simulink model "test12"  (R2024a)
settings: Solver=FixedStepAuto  StartTime=0.0  StopTime=30  FixedStep=0.001  MaxStep=1e-2  RelTol=1e-3
libraries: fl_lib x21, nesl_utility x14, sdl_lib x8, simulink x4
(part 1 of 2)
settings Model: DataDictionary=test4.sldd  Creator=18311  LastModifiedBy=18311

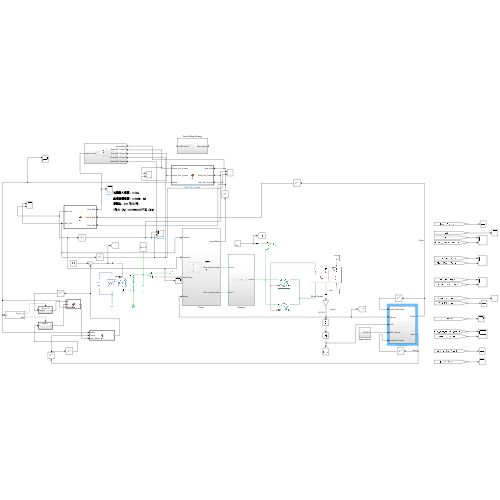
[thumbnail: Simulink's stored preview of the top-level diagram]
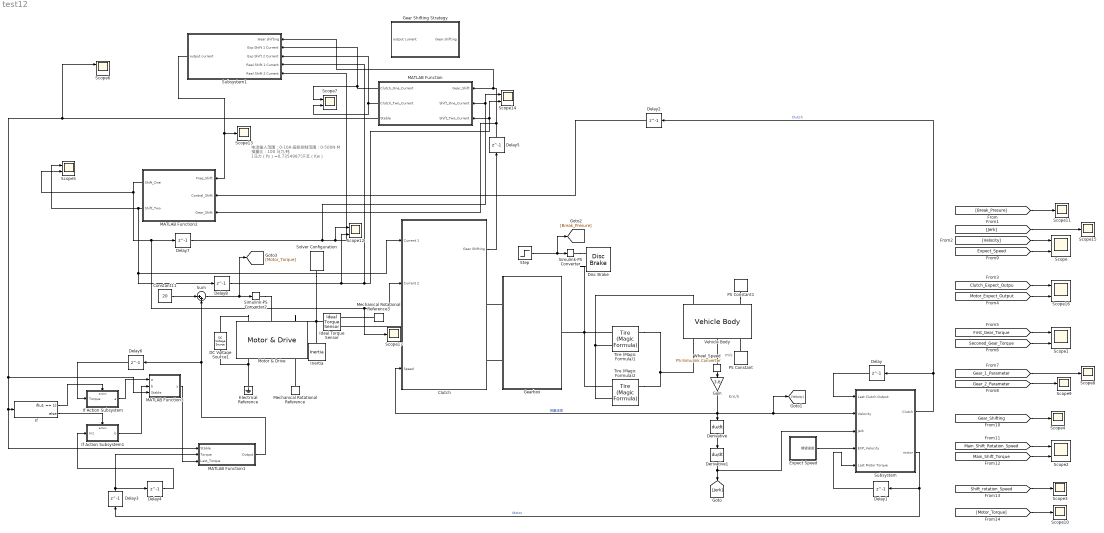
== system test12 ==
  note: Km/h
  note: m/s
  note: 电流输入范围：0-10A
      | 扭矩控制范围：0-500N·M
      | 推重比：100 马力/吨
      | 1马力（Ps）=0.73549875千瓦（Kw）
  Clutch : Subsystem
      settings: PortSchema="{\"entries\":[{\"content\":{\"sides\":[{\"content\":{\"connectorIds\":[\"In1\",\"In2\",\"LConn1\",\"In3\"]},\"type\":\"ConnectorPlacement.EquallySpacedRectSide\",\"uuid\":\"056ad525-3a8f-4273-b105-de9e991d8580\"},{\"content\":{\"connectorIds\":[\"Out1\",\"RConn1\",\"RConn2\"],\"side\":\"RIGHT\"},\"type\":\"ConnectorPlacement.EquallySpacedRectSide\",\"uuid\":\"78f39029-2d72-4f9a-95da-9e6af56cb8b6\"},{\"content\":{\"side\":\"TOP\"},\"type\":\"ConnectorPlacement.EquallySpacedRectSide\",\"uuid\":\"380b0431-6fdd-4cff-97a6-25de2baed91e\"}]},\"type\":\"ConnectorPlacement.EquallySpacedConnector\",\"uuid\":\"d5c6ad5a-c539-4d45-a449-cd47a7a8a4ab\"}],\"packageUris\":[\"http://schema.mathworks.com/mf0/Connector/R2020b\"],\"version\":\"1.0\"}"
  Constant11 : Constant  Value=20
  DC Voltage Source1 : fl_lib/Electrical/Electrical Sources/DC Voltage Source  v0=220 V
  Delay{,1..8} (9 alike) : Delay  DelayLength=1  InitialCondition=0
  Derivative : Derivative
  Derivative1 : Derivative
  Disc Brake : sdl_lib/Brakes & Detents/Rotational/Disc Brake  r_mean=150 mm  bore=10 mm  n_pads=2  enable_faults=simscape.enum.onoff.off  faulted_pressure=0 bar  thermal_port=simscape.enum.thermaleffects.omit  mu_static=0.9  mu_coulomb=0.7  temperature_TLU=[280, 300, 320] K  mu_static_TLU=[.9, .8, .7]  mu_coulomb_TLU=[.8, .7, .6]  brkwy_vel=0.1 rad/s  visc_coef=0 N*m*s/rad  thermal_mass=50 kJ/K  temperature_specify=off  temperature_priority=High  temperature=300 K  temperature_nominal_specify=off  temperature_nominal_value=1  temperature_nominal_unit=K
  Electrical Reference : fl_lib/Electrical/Electrical Elements/Electrical Reference
  Expect Speed : Subsystem
  Gain : Gain  Gain=3.6
  Gear Shifting Strategy : Subsystem
  Gearbox : Subsystem
  Ideal Torque Sensor : fl_lib/Mechanical/Mechanical Sensors/Ideal Torque Sensor
  If : If  IfExpression=u1 == 1
  If Action Subsystem : Subsystem  TreatAsAtomicUnit=on
  If Action Subsystem1 : Subsystem  TreatAsAtomicUnit=on
  Inertia : fl_lib/Mechanical/Rotational Elements/Inertia  inertia=0.01 kg*m^2  num_ports=foundation.enum.numPorts2.one  w_specify=off  w_priority=High  w=0 rad/s  w_nominal_specify=off  w_nominal_value=1  w_nominal_unit=rad/s  t_specify=off  t_priority=None  t=0 N*m  t_nominal_specify=off  t_nominal_value=1  t_nominal_unit=N*m
  MATLAB Function : MATLAB Function  TreatAsAtomicUnit=on
  MATLAB Function1 : MATLAB Function  TreatAsAtomicUnit=on
  MATLAB Function2 : MATLAB Function  TreatAsAtomicUnit=on
  MATLAB Function3 : MATLAB Function  TreatAsAtomicUnit=on
  Mechanical Rotational Reference : fl_lib/Mechanical/Rotational Elements/Mechanical Rotational Reference
  Mechanical Rotational Reference3 : fl_lib/Mechanical/Rotational Elements/Mechanical Rotational Reference
  Motor & Drive : sdl_lib/Engines & Motors/Motor & Drive  torque_max=200 N*m  power_max=73.549875 kW  Tc=0.02 s  eff=100  w_eff=4000 rpm  T_eff=200 N*m  thermal_port=simscape.enum.thermaleffects.omit  thermal_mass=100 J/K  temperature_specify=off  temperature_priority=High  temperature=300 K  temperature_nominal_specify=off  temperature_nominal_value=1  temperature_nominal_unit=K
      settings: InternalSimscapePortConfiguration="{\"Bottom\":[],\"Left\":[{\"id\":\"Vp\",\"label\":\"+\",\"type\":\"foundation.electrical.electrical\"},{\"id\":\"Tr\",\"label\":\"Tr\",\"type\":\"input\"},{\"id\":\"R\",\"label\":\"R\",\"type\":\"foundation.mechanical.rotational.rotational\"}],\"Right\":[{\"id\":\"Vm\",\"label\":\"-\",\"type\":\"foundation.electrical.electrical\"},{\"id\":\"Omega\",\"label\":\"w\",\"type\":\"output\"},{\"id\":\"C\",\"label\":\"C\",\"type\":\"foundation.mechanical.rotational.rotational\"}],\"Top\":[]}"
  PS Constant : fl_lib/Physical Signals/Sources/PS Constant  constant=0
  PS Constant1 : fl_lib/Physical Signals/Sources/PS Constant  constant=0
  Scope{,1..2,5..7,12,14,16} (9 alike) : Scope  NumInputPorts=2
  Scope{3..4,8..11,13,15,17} (9 alike) : Scope
  Simulink-PS Converter : nesl_utility/Simulink-PS Converter  PhysicalDomain=network_engine_domain  SubClassName=ps_input  LeftPortType=input  RightPortType=output  PseudoPeriodic=off  Frequencies=[]  NoiseDistribution=none  NoiseParameters=[]  Unit=1  AffineConversion=off  FilteringAndDerivatives=provide  SimscapeFilterOrder=1  InputFilterTimeConstant=0.001  UdotUserProvided=0
  Simulink-PS Converter2 : nesl_utility/Simulink-PS Converter  PhysicalDomain=network_engine_domain  SubClassName=ps_input  LeftPortType=input  RightPortType=output  PseudoPeriodic=off  Frequencies=[]  NoiseDistribution=none  NoiseParameters=[]  Unit=1  AffineConversion=off  FilteringAndDerivatives=provide  SimscapeFilterOrder=1  InputFilterTimeConstant=0.001  UdotUserProvided=0
  Solver Configuration : nesl_utility/Solver Configuration  PhysicalDomain=network_engine_domain  SubClassName=solver  LeftPortType=input  RightPortType=generic  Tones=[]  Harmonics=[]  SimulateNoise=off  Profile=off  UseLocalSampling=off  EnableSwitchedLinearOptims=on  FrequencyDomain=off  UseCCode=off  RelTol=0.001  AbsTol=0.001  MinStep=1e-09  ToWorkspace=off  RevertToSquareIcSolve=off  NumHomotopyIterations=100  PhasorMode=off  PhasorModeNumHarmonics=1  ConsistencySolver=NEWTON_XTOL_AFTER_FTOL  IndexReductionMethod=DerivativeReplacement  DoDC=off  ResidualTolerance=1e-09  ConsistencyTolSource=GLOBAL  ConsistencyAbsTol=0.001  ConsistencyRelTol=0.001  ConsistencyTolFactor=0.001  UseLocalSolver=off  LocalSolverChoice=NE_BACKWARD_EULER_ADVANCER  ResolveIndetEquations=on  FunctionEvalNumThread=1  LocalSolverSampleTime=0.001  DoFixedCost=off  MaxNonlinIter=3  MaxModeIter=2  ComputeImpulses=off  ImpulseIterations=2  LinearAlgebra=auto  LinearAlgebraNumThread=0  EquationFormulation=NE_TIME_EF  DelaysMemoryBudget=1024  AutomaticFiltering=on  FilteringTimeConstant=0.001  PartitionStorageMethod=AS_NEEDED  PartitionMemoryBudget=1024  PartitionMethod=ROBUST  MultibodyUseLocalSolver=off  MultibodyLocalSolverChoice=ODE1  MultibodyLocalSolverSampleTime=0.001
  Step : Step  Time=20  After=150  SampleTime=0
  Subsystem : Subsystem
  Subsystem1 : Subsystem
  Sum : Sum  Inputs=|++
  Tire (Magic Formula)1 : sdl_lib/Tires & Vehicles/Tire (Magic Formula)  parameterization=sdl.enum.magic_tire_model.peak  F_z1=2500 N  F_x1=3500 N  kappa1=10  B_m=10  C_m=1.9  D_m=1  E_m=0.97  fz0=4000 N  p_Cx=1.685  p_Dx=[1.21, -.037]  p_Ex=[.344, .095, -.02, 0]  p_Kx=[21.51, -.163, .245]  p_Hx=[-.002, .002]  p_Vx=[0, 0]  rolling_radius_model=sdl.enum.RollingRadiusParameterization.Constant  r_e=0.3 m  r_0=0.3 m  breff=8.39  dreff=0.26  freff=0.074  q_re0=0.99  q_v1=0.008  longvl=17 m/s  cz=5e5 N/m  model_resistance=true  resistance_model=sdl.enum.rollingResistanceParameterization.constant  coeff=0.015  p_tire=250e3 Pa  alpha=-0.003  beta=0.97  coeff_a=84e-4  coeff_b=6.2e-4 s/m  coeff_c=1.6e-4 s^2/m^2  p_tire0=240e3 Pa  fz0_resistance=4000 N  vH0=16 m/s  q_Sy=[.0082, 0, .0014, .001, 0, 0, 1.08, -.5]  v_thr=0.001 m/s  enable_scaling_coefficients=false  lfzO=1  lcx=1  lmux=1  lex=1  lkx=1  lhx=1  lvx=1  lmy=1  model_compliance=sdl.enum.compliance.off  stiffness=1e6 N/m  damping=1000 N*s/m  model_inertia=sdl.enum.model_inertia.off  inertia=1 kg*m^2  initial_velocity=0 rad/s  vxlow=1 m/s  v_tr_thr=0.1 m/s  kpumin=-1.5  kpumax=1.5
  Tire (Magic Formula)2 : sdl_lib/Tires & Vehicles/Tire (Magic Formula)  parameterization=sdl.enum.magic_tire_model.peak  F_z1=2500 N  F_x1=3000 N  kappa1=10  B_m=10  C_m=1.9  D_m=1  E_m=0.97  fz0=4000 N  p_Cx=1.685  p_Dx=[1.21, -.037]  p_Ex=[.344, .095, -.02, 0]  p_Kx=[21.51, -.163, .245]  p_Hx=[-.002, .002]  p_Vx=[0, 0]  rolling_radius_model=sdl.enum.RollingRadiusParameterization.Constant  r_e=0.3 m  r_0=0.3 m  breff=8.39  dreff=0.26  freff=0.074  q_re0=0.99  q_v1=0.008  longvl=17 m/s  cz=5e5 N/m  model_resistance=true  resistance_model=sdl.enum.rollingResistanceParameterization.constant  coeff=0.015  p_tire=250e3 Pa  alpha=-0.003  beta=0.97  coeff_a=84e-4  coeff_b=6.2e-4 s/m  coeff_c=1.6e-4 s^2/m^2  p_tire0=240e3 Pa  fz0_resistance=4000 N  vH0=16 m/s  q_Sy=[.0082, 0, .0014, .001, 0, 0, 1.08, -.5]  v_thr=0.001 m/s  enable_scaling_coefficients=false  lfzO=1  lcx=1  lmux=1  lex=1  lkx=1  lhx=1  lvx=1  lmy=1  model_compliance=sdl.enum.compliance.off  stiffness=1e6 N/m  damping=1000 N*s/m  model_inertia=sdl.enum.model_inertia.off  inertia=1 kg*m^2  initial_velocity=0 rad/s  vxlow=1 m/s  v_tr_thr=0.1 m/s  kpumin=-1.5  kpumax=1.5
  Vehicle Body : sdl_lib/Tires & Vehicles/Vehicle Body  mass=1000 kg  n_w=1  x_f=1.4 m  x_r=1.6 m  y_c=0.5 m  mass_var=simscape.enum.onoff.off  g=9.81 m/s^2  liftoff_warning=simscape.enum.onoff.off  area=3 m^2  Cd=0.4  rho=1.18 kg/m^3  model_pitch=simscape.enum.onoff.off  inertia=4000 kg*m^2  suspension_model=sdl.enum.linearTLU.linear  k_f=1e4 N/m  b_f=1e4 N*s/m  k_r=1e4 N/m  b_r=1e4 N*s/m  k_f_TLU=[-2000, -1000, 0, 1000, 2000] N  x_f_TLU=[-.4, -.2, 0, .2, .4] m  b_f_TLU=[-200, -100, 0, 100, 200] N  v_f_TLU=[-4, -2, 0, 2, 4] m/s  k_r_TLU=[-2000, -1000, 0, 1000, 2000] N  x_r_TLU=[-.4, -.2, 0, .2, .4] m  b_r_TLU=[-200, -100, 0, 100, 200] N  v_r_TLU=[-4, -2, 0, 2, 4] m/s  interp_method=simscape.enum.interpolation.linear  extrap_method=simscape.enum.extrapolation.linear  model_hardstop=simscape.enum.onoff.off  upper_bound_f=.25 m  lower_bound_f=-.25 m  stop_k_f=1e6 N/m  stop_b_f=150 N*s/m  upper_bound_r=.25 m  lower_bound_r=-.25 m  stop_k_r=1e6 N/m  stop_b_r=150 N*s/m  initial_pitch=0 rad  initial_pitch_rate=0 rad/s  v_specify=off  v_priority=High  v=0 m/s  v_nominal_specify=off  v_nominal_value=1  v_nominal_unit=m/s
  Wheel_Speed : nesl_utility/PS-Simulink Converter  PhysicalDomain=network_engine_domain  SubClassName=ps_output  LeftPortType=input  RightPortType=output  PseudoPeriodic=off  Frequencies=[]  VectorFormat=inherit  Unit=inherit  AffineConversion=off
  wires:
  Wheel_Speed/1 -> Gain/1
  Derivative/1 -> Derivative1/1
  Constant11/1 -> Sum/1
  Sum/1 -> [Motor_Torque], Simulink-PS Converter2/1
  Subsystem/2(motor) -> Delay1/1, Delay3/1  "Motor"
  Subsystem/1(Clutch) -> Delay2/1, Delay/1  "Clutch"
  Gain/1 -> Derivative/1, [Velocity], Subsystem/2(Velocity), Clutch/3(Speed)  "测量速度"
  Clutch/1(Gear Shifting) -> Delay5/1
  Expect Speed/1(期望速度) -> Subsystem/4(EXP_Velocity)
  Delay/1 -> Subsystem/1(Last Clutch Output)
  Delay1/1 -> Subsystem/5(Last Motor Torque)
  Derivative1/1 -> [Jerk], Subsystem/3(Jerk)
  [Velocity] -> Scope/1
  [Expect_Speed] -> Scope/2
  [First_Gear_Torque] -> Scope1/1
  [Seconed_Gear_Torque] -> Scope1/2
  [Main_Shift_Torque] -> Scope2/2
  [Main_Shift_Rotation_Speed] -> Scope2/1
  [Shift_rotation_Speed] -> Scope3/1
  Delay5/1 -> MATLAB Function2/3(Gear_Shift), Subsystem1/1(Gear shifting), MATLAB Function/1(Gear_Shift)
  If/1 -> If Action Subsystem/Action
  If/2 -> If Action Subsystem1/Action
  MATLAB Function/3(Stable) -> Scope6/1, MATLAB Function3/3(Stable), MATLAB Function1/1(Stable), If/1
  Delay3/1 -> MATLAB Function1/2(Torque), Delay4/1
  MATLAB Function1/1(Output) -> Delay6/1, Sum/2
  Delay4/1 -> If Action Subsystem1/1(In1)
  Delay6/1 -> If Action Subsystem/1(Torque)
  MATLAB Function3/1(y) -> MATLAB Function1/3(Last_Torque)
  If Action Subsystem/1(a) -> MATLAB Function3/1(a)
  If Action Subsystem1/1(b) -> MATLAB Function3/2(b)
  MATLAB Function/1(Clutch_One_Current) -> Subsystem1/2(Exp Shift 1 Current), Scope7/1
  MATLAB Function/2(Clutch_Two_Current) -> Subsystem1/3(Exp Shift 2 Current), Scope7/2
  Delay2/1 -> MATLAB Function2/2(Contral_Shift)
  Subsystem1/1(output current) -> Scope13/1, MATLAB Function2/1(Free_Shift)
  MATLAB Function2/1(Shift_One) -> Scope5/2, Clutch/2(Current 2), Scope17/1, Delay7/1
  MATLAB Function2/2(Shift_Two) -> Scope5/1, Delay8/1, Clutch/1(Current 1)
  [Gear_Shifting] -> Scope4/1
  Delay7/1 -> Subsystem1/5(Real Shift 2 Current), Scope12/1, Scope14/1, MATLAB Function/2(Shift_One_Current)
  Delay8/1 -> Subsystem1/4(Real Shift 1 Current), Scope14/2, MATLAB Function/3(Shift_Two_Current), Scope12/2
  [Gear_1_Parameter] -> Scope8/1
  [Gear_2_Parameter] -> Scope9/1
  [Motor_Torque] -> Scope10/1
  [Break_Presure] -> Scope11/1
  Step/1 -> [Break_Presure], Simulink-PS Converter/1
  [Jerk] -> Scope15/1
  [Clutch_Expect_Outpu] -> Scope16/1
  [Motor_Expect_Output] -> Scope16/2
  connections:
  Motor & Drive/LConn1 -- DC Voltage Source1/LConn1
  Electrical Reference/LConn1 -- DC Voltage Source1/RConn1 -- Motor & Drive/RConn1
  Mechanical Rotational Reference/LConn1 -- Motor & Drive/RConn3
  Inertia/LConn1 -- Motor & Drive/LConn3 -- Solver Configuration/RConn1 -- Ideal Torque Sensor/LConn1
  PS Constant/RConn1 -- Vehicle Body/LConn3
  PS Constant1/RConn1 -- Vehicle Body/RConn3
  Clutch/LConn1 -- Ideal Torque Sensor/RConn2
  Wheel_Speed/LConn1 -- Vehicle Body/LConn2
  Simulink-PS Converter2/RConn1 -- Motor & Drive/LConn2
  Tire (Magic Formula)1/RConn2 -- Tire (Magic Formula)2/RConn2 -- Vehicle Body/LConn1
  Tire (Magic Formula)1/LConn1 -- Tire (Magic Formula)2/LConn1 -- Vehicle Body/RConn1
  Mechanical Rotational Reference3/LConn1 -- Ideal Torque Sensor/RConn1
  Simulink-PS Converter/RConn1 -- Disc Brake/LConn1
  Disc Brake/LConn2 -- Tire (Magic Formula)1/LConn2 -- Tire (Magic Formula)2/LConn2 -- Gearbox/RConn1
  Gearbox/LConn1 -- Clutch/RConn1
  Gearbox/LConn2 -- Clutch/RConn2

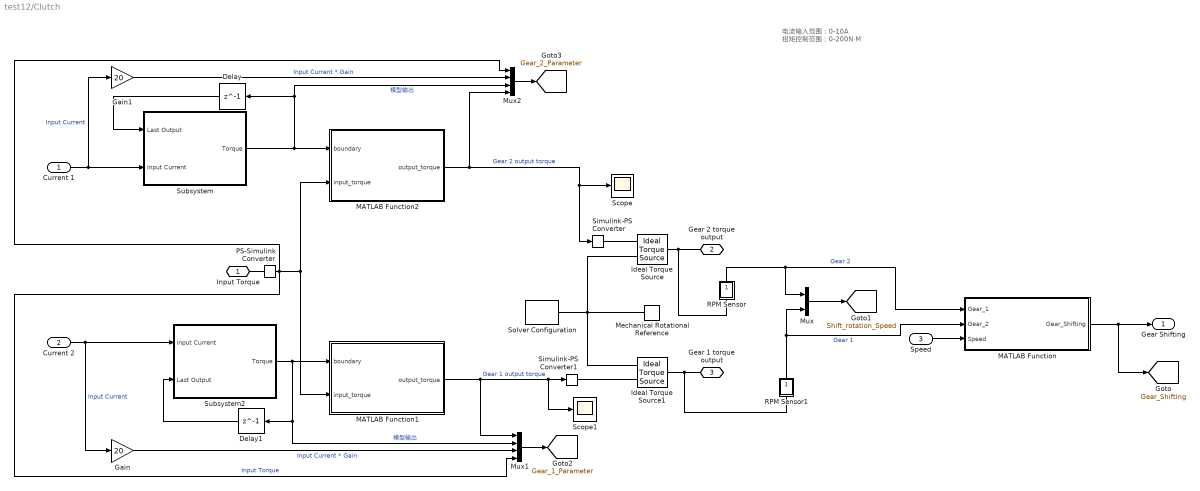
== system test12/Clutch ==
  note: 电流输入范围：0-10A
      | 扭矩控制范围：0-200N·M
  Current 1 : Inport
  Current 2 : Inport  Port=2
  Speed : Inport  Port=3
  Delay : Delay  DelayLength=1  InitialCondition=0
  Delay1 : Delay  DelayLength=1  InitialCondition=0
  Gain : Gain  Gain=20
  Gain1 : Gain  Gain=20
  Ideal Torque Source : fl_lib/Mechanical/Mechanical Sources/Ideal Torque Source
  Ideal Torque Source1 : fl_lib/Mechanical/Mechanical Sources/Ideal Torque Source
  MATLAB Function : MATLAB Function  TreatAsAtomicUnit=on
  MATLAB Function1 : MATLAB Function  TreatAsAtomicUnit=on
  MATLAB Function2 : MATLAB Function  TreatAsAtomicUnit=on
  Mechanical Rotational Reference : fl_lib/Mechanical/Rotational Elements/Mechanical Rotational Reference
  Mux : Mux  Inputs=2
  Mux1 : Mux
  Mux2 : Mux
  PS-Simulink Converter : nesl_utility/PS-Simulink Converter  PhysicalDomain=network_engine_domain  SubClassName=ps_output  LeftPortType=input  RightPortType=output  PseudoPeriodic=off  Frequencies=[]  VectorFormat=inherit  Unit=inherit  AffineConversion=off
  RPM Sensor : Subsystem
      mask Display: disp('S')
  RPM Sensor1 : Subsystem
      mask Display: disp('S')
  Scope : Scope
  Scope1 : Scope
  Simulink-PS Converter : nesl_utility/Simulink-PS Converter  PhysicalDomain=network_engine_domain  SubClassName=ps_input  LeftPortType=input  RightPortType=output  PseudoPeriodic=off  Frequencies=[]  NoiseDistribution=none  NoiseParameters=[]  Unit=1  AffineConversion=off  FilteringAndDerivatives=provide  SimscapeFilterOrder=1  InputFilterTimeConstant=0.001  UdotUserProvided=0
  Simulink-PS Converter1 : nesl_utility/Simulink-PS Converter  PhysicalDomain=network_engine_domain  SubClassName=ps_input  LeftPortType=input  RightPortType=output  PseudoPeriodic=off  Frequencies=[]  NoiseDistribution=none  NoiseParameters=[]  Unit=1  AffineConversion=off  FilteringAndDerivatives=provide  SimscapeFilterOrder=1  InputFilterTimeConstant=0.001  UdotUserProvided=0
  Solver Configuration : nesl_utility/Solver Configuration  PhysicalDomain=network_engine_domain  SubClassName=solver  LeftPortType=input  RightPortType=generic  Tones=[]  Harmonics=[]  SimulateNoise=off  Profile=off  UseLocalSampling=off  EnableSwitchedLinearOptims=on  FrequencyDomain=off  UseCCode=off  RelTol=0.001  AbsTol=0.001  MinStep=1e-09  ToWorkspace=off  RevertToSquareIcSolve=off  NumHomotopyIterations=100  PhasorMode=off  PhasorModeNumHarmonics=1  ConsistencySolver=NEWTON_XTOL_AFTER_FTOL  IndexReductionMethod=DerivativeReplacement  DoDC=off  ResidualTolerance=1e-09  ConsistencyTolSource=GLOBAL  ConsistencyAbsTol=0.001  ConsistencyRelTol=0.001  ConsistencyTolFactor=0.001  UseLocalSolver=off  LocalSolverChoice=NE_BACKWARD_EULER_ADVANCER  ResolveIndetEquations=on  FunctionEvalNumThread=1  LocalSolverSampleTime=0.001  DoFixedCost=off  MaxNonlinIter=3  MaxModeIter=2  ComputeImpulses=off  ImpulseIterations=2  LinearAlgebra=auto  LinearAlgebraNumThread=0  EquationFormulation=NE_TIME_EF  DelaysMemoryBudget=1024  AutomaticFiltering=on  FilteringTimeConstant=0.001  PartitionStorageMethod=AS_NEEDED  PartitionMemoryBudget=1024  PartitionMethod=ROBUST  MultibodyUseLocalSolver=off  MultibodyLocalSolverChoice=ODE1  MultibodyLocalSolverSampleTime=0.001
  Subsystem : Subsystem  mask{c=-2, k=20, d=0.6, alpha=-37.209}
  Subsystem2 : Subsystem  mask{c=-2, k=20, d=0.6, alpha=-37.209}
  Input Torque : PMIOPort  Side=Left
  Gear 2 torque output : PMIOPort  Port=2  Side=Right
  Gear 1 torque output : PMIOPort  Port=3  Side=Right
  Gear Shifting : Outport
  tag scope: Gear_1_Parameter=global, Gear_2_Parameter=global, Gear_Shifting=global, Shift_rotation_Speed=global
  wires:
  Current 2/1 -> Gain/1, Subsystem2/1(Input Current)  "Input Current"
  MATLAB Function1/1(output_torque) -> Mux1/1, Scope1/1, Simulink-PS Converter1/1  "Gear 1 output torque"
  MATLAB Function2/1(output_torque) -> Mux2/4, Scope/1, Simulink-PS Converter/1  "Gear 2 output torque"
  PS-Simulink Converter/1 -> Mux2/1, Mux1/4, MATLAB Function2/2(input_torque), MATLAB Function1/2(input_torque)  "Input Torque"
  RPM Sensor/1(rpm) -> Mux/1, MATLAB Function/1(Gear_1)  "Gear 2"
  Subsystem2/1(Torque) -> Mux1/2, Delay1/1, MATLAB Function1/1(boundary)  "模型输出"
  RPM Sensor1/1(rpm) -> Mux/2, MATLAB Function/2(Gear_2)  "Gear 1"
  Subsystem/1(Torque) -> Mux2/3, Delay/1, MATLAB Function2/1(boundary)  "模型输出"
  Speed/1 -> MATLAB Function/3(Speed)
  MATLAB Function/1(Gear_Shifting) -> [Gear_Shifting], Gear Shifting/1
  Mux/1 -> [Shift_rotation_Speed]
  Delay1/1 -> Subsystem2/2(Last Output)
  Current 1/1 -> Gain1/1, Subsystem/2(Input Current)  "Input Current"
  Delay/1 -> Subsystem/1(Last Output)
  Mux1/1 -> [Gear_1_Parameter]
  Mux2/1 -> [Gear_2_Parameter]
  Gain/1 -> Mux1/3  "Input Current * Gain"
  Gain1/1 -> Mux2/2  "Input Current * Gain"
  connections:
  Input Torque/RConn1 -- PS-Simulink Converter/LConn1
  Ideal Torque Source/RConn2 -- Ideal Torque Source1/RConn2 -- Mechanical Rotational Reference/LConn1 -- Solver Configuration/RConn1
  Ideal Torque Source/LConn1 -- RPM Sensor/LConn1 -- Gear 2 torque output/RConn1
  Ideal Torque Source1/LConn1 -- RPM Sensor1/LConn1 -- Gear 1 torque output/RConn1
  Ideal Torque Source/RConn1 -- Simulink-PS Converter/RConn1
  Ideal Torque Source1/RConn1 -- Simulink-PS Converter1/RConn1

== system test12/Expect Speed ==
  Add : Sum  Inputs=+++
  Constant : Constant  Value=80
  Constant1 : Constant  Value=0
  Ramp : simulink/Sources/Ramp  slope=8  start=0  InitialOutput=0
  Ramp1 : simulink/Sources/Ramp  slope=-8  start=10  InitialOutput=0
  Ramp2 : simulink/Sources/Ramp  slope=-8  start=20  InitialOutput=0
  Saturation Dynamic : simulink/Discontinuities/Saturation Dynamic  OutMin=[]  OutMax=[]  OutDataTypeStr=Inherit: Same as second input  OutDataType=fixdt(1, 16)  OutScaling=2^-10  DoSatur=off
  期望速度 : Outport
  tag scope: Expect_Speed=global
  wires:
  Constant1/1 -> Saturation Dynamic/3
  Constant/1 -> Saturation Dynamic/1
  Ramp/1 -> Add/1
  Ramp2/1 -> Add/3
  Add/1 -> Saturation Dynamic/2
  Ramp1/1 -> Add/2
  Saturation Dynamic/1 -> 期望速度/1, [Expect_Speed]  "期望速度"

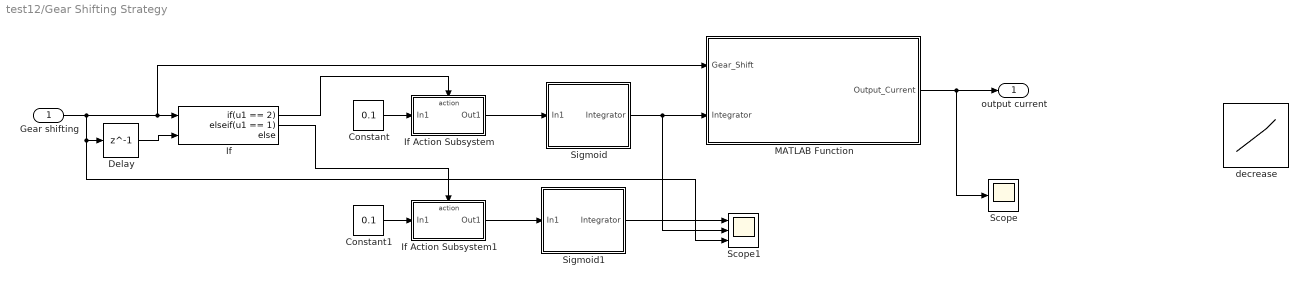
== system test12/Gear Shifting Strategy ==
  Gear shifting : Inport
  Constant : Constant  Value=0.1
  Constant1 : Constant  Value=0.1
  Delay : Delay  DelayLength=1  InitialCondition=0
  If : If  NumInputs=2  IfExpression=u1 == 2  ElseIfExpressions=u1 == 1
  If Action Subsystem : Subsystem  TreatAsAtomicUnit=on
  If Action Subsystem1 : Subsystem  TreatAsAtomicUnit=on
  MATLAB Function : MATLAB Function  TreatAsAtomicUnit=on
  Scope : Scope
  Scope1 : Scope  NumInputPorts=3
  Sigmoid : Subsystem
  Sigmoid1 : Subsystem
  decrease : Lookup_n-D  NumberOfTableDimensions=1  BreakpointsForDimension1=[0:1:10]  Table=10*1./(1+exp(-[0:1:10]+5))  InternalRulePriority=Speed  RndMeth=Simplest
  output current : Outport
  wires:
  Gear shifting/1 -> MATLAB Function/1(Gear_Shift), If/1, Scope1/3, Delay/1
  If/1 -> If Action Subsystem/Action
  Constant/1 -> If Action Subsystem/1(In1)
  If Action Subsystem/1(Out1) -> Sigmoid/1(In1)
  MATLAB Function/1(Output_Current) -> Scope/1, output current/1
  Sigmoid/1(Integrator) -> Scope1/2, MATLAB Function/2(Integrator)
  Constant1/1 -> If Action Subsystem1/1(In1)
  Delay/1 -> If/2
  If/2 -> If Action Subsystem1/Action
  Sigmoid1/1(Integrator) -> Scope1/1
  If Action Subsystem1/1(Out1) -> Sigmoid1/1(In1)

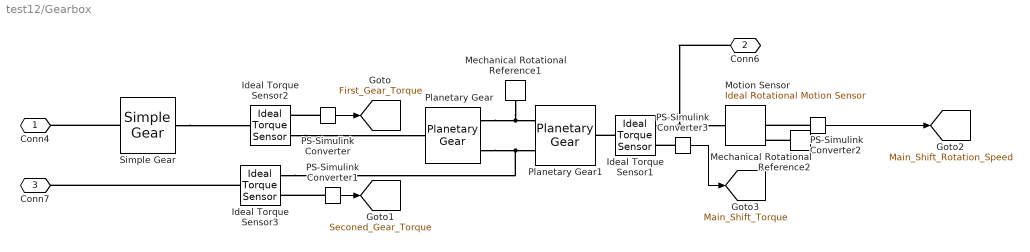
== system test12/Gearbox ==
  Ideal Torque Sensor1 : fl_lib/Mechanical/Mechanical Sensors/Ideal Torque Sensor
  Ideal Torque Sensor2 : fl_lib/Mechanical/Mechanical Sensors/Ideal Torque Sensor
  Ideal Torque Sensor3 : fl_lib/Mechanical/Mechanical Sensors/Ideal Torque Sensor
  Mechanical Rotational Reference1 : fl_lib/Mechanical/Rotational Elements/Mechanical Rotational Reference
  Mechanical Rotational Reference2 : fl_lib/Mechanical/Rotational Elements/Mechanical Rotational Reference
  Motion Sensor : fl_lib/Mechanical/Mechanical Sensors/Ideal Rotational Motion Sensor  reference=foundation.enum.MeasurementReference.difference  acceleration_port=false  velocity_port=true  position_port=true  wrap_angle=simscape.enum.onoff.off  offset=0 rad
  PS-Simulink Converter{,1..3} (4 alike) : nesl_utility/PS-Simulink Converter  PhysicalDomain=network_engine_domain  SubClassName=ps_output  LeftPortType=input  RightPortType=output  PseudoPeriodic=off  Frequencies=[]  VectorFormat=inherit  Unit=inherit  AffineConversion=off
  Planetary Gear : sdl_lib/Gears/Planetary Gear  rs_ratio=3  friction_model=sdl.enum.gear_friction.none  efficiency=[.96, .98]  temperature_TLU=[280, 300, 320] K  efficiency_sp_TLU=[.95, .9, .85]  efficiency_rp_TLU=[.95, .9, .85]  pwr_thr=[.001, .001] W  mu_visc=[0, 0] N*m*s/rad  model_inertia=simscape.enum.onoff.off  planet_inertia=0.001 kg*m^2  thermal_mass=50 J/K  T_init=300 K
  Planetary Gear1 : sdl_lib/Gears/Planetary Gear  rs_ratio=6  friction_model=sdl.enum.gear_friction.none  efficiency=[.96, .98]  temperature_TLU=[280, 300, 320] K  efficiency_sp_TLU=[.95, .9, .85]  efficiency_rp_TLU=[.95, .9, .85]  pwr_thr=[.001, .001] W  mu_visc=[0, 0] N*m*s/rad  model_inertia=simscape.enum.onoff.off  planet_inertia=0.001 kg*m^2  thermal_mass=50 J/K  T_init=300 K
  Simple Gear : sdl_lib/Gears/Simple Gear  ratio=3  rotation_direction=sdl.enum.shaftOutputDirection.same  enable_faults=simscape.enum.onoff.off  efficiency_fault=0.05  fault_angles=pi / 12 rad  friction_model=sdl.enum.gear_efficiencies_load.off  T_noload=0.1 N*m  T_nom=5 N*m  efficiency_nom=0.8  efficiency=0.8  temperature_TLU=[280, 300, 320] K  load_TLU=[1, 5, 10] N*m  efficiency_TLU=[.95, .9, .85]  efficiency_TLU2=[.85, .8, .75; .95, .9, .85; .85, .8, .7]  w_thr=0.01 rad/s  pwr_thr=0.001 W  enable_backlash=false  hardstop_model=simscape.enum.hardstop.smooth  backlash_distance=1e-3 mm  r_base=0.1 m  transition=1e-4 mm  backlash_stiffness=1e6 N/m  backlash_damping=1e3 N*s/m  coeff_rest=0.7  v_tol=0.001 m/s  f_tol=0.001 N  mu_visc=[0, 0] N*m*s/rad  thermal_mass=50 J/K  temperature_specify=off  temperature_priority=High  temperature=300 K  temperature_nominal_specify=off  temperature_nominal_value=1  temperature_nominal_unit=K  x_backlash_specify=off  x_backlash_priority=None  x_backlash=0 mm  x_backlash_nominal_specify=off  x_backlash_nominal_value=1  x_backlash_nominal_unit=mm  f_hardstop_specify=off  f_hardstop_priority=None  f_hardstop=0 N  f_hardstop_nominal_specify=off  f_hardstop_nominal_value=1  f_hardstop_nominal_unit=N  v_backlash_specify=off  v_backlash_priority=None  v_backlash=0 m/s  v_backlash_nominal_specify=off  v_backlash_nominal_value=1  v_backlash_nominal_unit=m/s
  Conn4 : PMIOPort  Side=Left
  Conn6 : PMIOPort  Port=2  Side=Right
  Conn7 : PMIOPort  Port=3  Side=Left
  tag scope: First_Gear_Torque=global, Main_Shift_Rotation_Speed=global, Main_Shift_Torque=global, Seconed_Gear_Torque=global
  wires:
  PS-Simulink Converter/1 -> [First_Gear_Torque]
  PS-Simulink Converter1/1 -> [Seconed_Gear_Torque]
  PS-Simulink Converter2/1 -> [Main_Shift_Rotation_Speed]
  PS-Simulink Converter3/1 -> [Main_Shift_Torque]
  connections:
  Mechanical Rotational Reference2/LConn1 -- Motion Sensor/RConn1
  Planetary Gear/RConn1 -- Mechanical Rotational Reference1/LConn1 -- Planetary Gear1/RConn1
  Planetary Gear/RConn2 -- Ideal Torque Sensor3/RConn1 -- Planetary Gear1/RConn2
  Ideal Torque Sensor1/LConn1 -- Planetary Gear1/LConn1
  Ideal Torque Sensor1/RConn1 -- Conn6/RConn1 -- Motion Sensor/LConn1
  Ideal Torque Sensor2/RConn1 -- Planetary Gear/LConn1
  Simple Gear/RConn1 -- Ideal Torque Sensor2/LConn1
  Ideal Torque Sensor3/LConn1 -- Conn7/RConn1
  Simple Gear/LConn1 -- Conn4/RConn1
  PS-Simulink Converter1/LConn1 -- Ideal Torque Sensor3/RConn2
  PS-Simulink Converter/LConn1 -- Ideal Torque Sensor2/RConn2
  PS-Simulink Converter2/LConn1 -- Motion Sensor/RConn2
  PS-Simulink Converter3/LConn1 -- Ideal Torque Sensor1/RConn2

== system test12/If Action Subsystem ==
  Torque : Inport
  Action Port : ActionPort  InitializeStates=reset  ActionPortLabel=if(u1 == 1)
  a : Outport
  wires:
  Torque/1 -> a/1

== system test12/If Action Subsystem1 ==
  In1 : Inport
  Action Port : ActionPort  InitializeStates=reset  ActionPortLabel=else
  b : Outport
  wires:
  In1/1 -> b/1

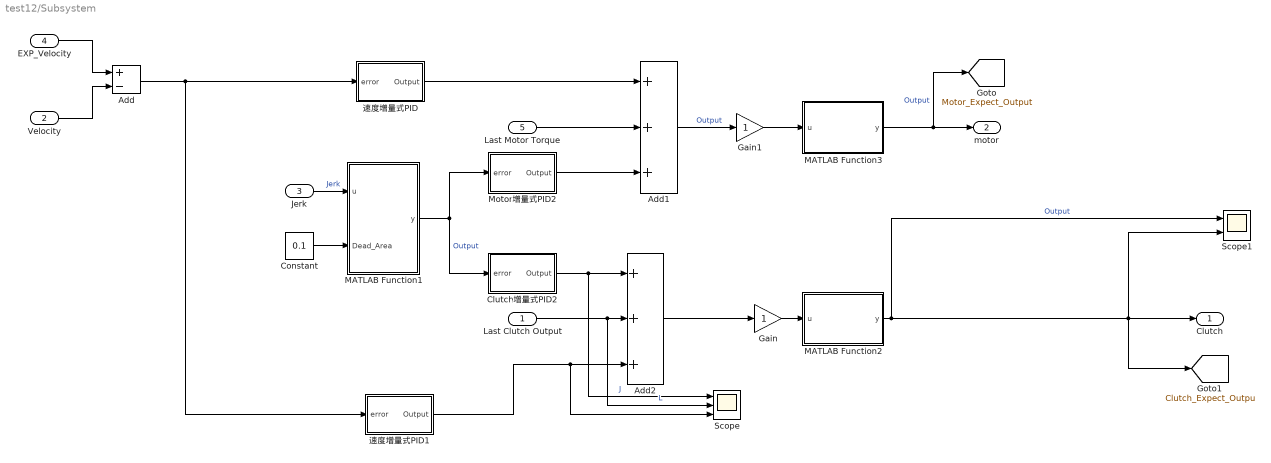
== system test12/Subsystem ==
  Last Clutch Output : Inport
  Velocity : Inport  Port=2
  Jerk : Inport  Port=3
  EXP_Velocity : Inport  Port=4
  Last Motor Torque : Inport  Port=5
  Add : Sum  Inputs=+-
  Add1 : Sum  Inputs=+++
  Add2 : Sum  Inputs=+++
  Clutch增量式PID2 : Subsystem  mask{Kp=0.0002, Ki=0, Kd=0.00001}
      mask DialogControl ParameterGroupVar Prompt: 参数
  Constant : Constant  Value=0.1
  Gain : Gain
  Gain1 : Gain
  MATLAB Function1 : MATLAB Function  TreatAsAtomicUnit=on
  MATLAB Function2 : MATLAB Function  TreatAsAtomicUnit=on
  MATLAB Function3 : MATLAB Function  TreatAsAtomicUnit=on
  Motor增量式PID2 : Subsystem  mask{Kp=0, Ki=0, Kd=0}
      mask DialogControl ParameterGroupVar Prompt: 参数
  Scope : Scope  NumInputPorts=3
  Scope1 : Scope  NumInputPorts=2
  速度增量式PID : Subsystem  mask{Kp=20, Ki=0.2, Kd=0}
      mask DialogControl ParameterGroupVar Prompt: 参数
  速度增量式PID1 : Subsystem  mask{Kp=2, Ki=0.1, Kd=0}
      mask DialogControl ParameterGroupVar Prompt: 参数
  Clutch : Outport
  motor : Outport  Port=2
  tag scope: Clutch_Expect_Outpu=global, Motor_Expect_Output=global
  wires:
  Jerk/1 -> MATLAB Function1/1(u)  "Jerk"
  MATLAB Function1/1(y) -> Clutch增量式PID2/1(error), Motor增量式PID2/1(error)  "Output"
  Constant/1 -> MATLAB Function1/2(Dead_Area)
  Add2/1 -> Gain/1
  Gain/1 -> MATLAB Function2/1(u)
  EXP_Velocity/1 -> Add/1
  Velocity/1 -> Add/2
  Motor增量式PID2/1(Output) -> Add1/3
  Last Motor Torque/1 -> Add1/2
  速度增量式PID/1(Output) -> Add1/1
  Clutch增量式PID2/1(Output) -> Scope/1, Add2/1  "J"
  Last Clutch Output/1 -> Scope/2, Add2/2  "L"
  Gain1/1 -> MATLAB Function3/1(u)
  Add1/1 -> Gain1/1  "Output"
  MATLAB Function3/1(y) -> [Motor_Expect_Output], motor/1  "Output"
  速度增量式PID1/1(Output) -> Scope/3, Add2/3
  Add/1 -> 速度增量式PID1/1(error), 速度增量式PID/1(error)
  MATLAB Function2/1(y) -> [Clutch_Expect_Outpu], Scope1/2, Clutch/1, Scope1/1  "Output"

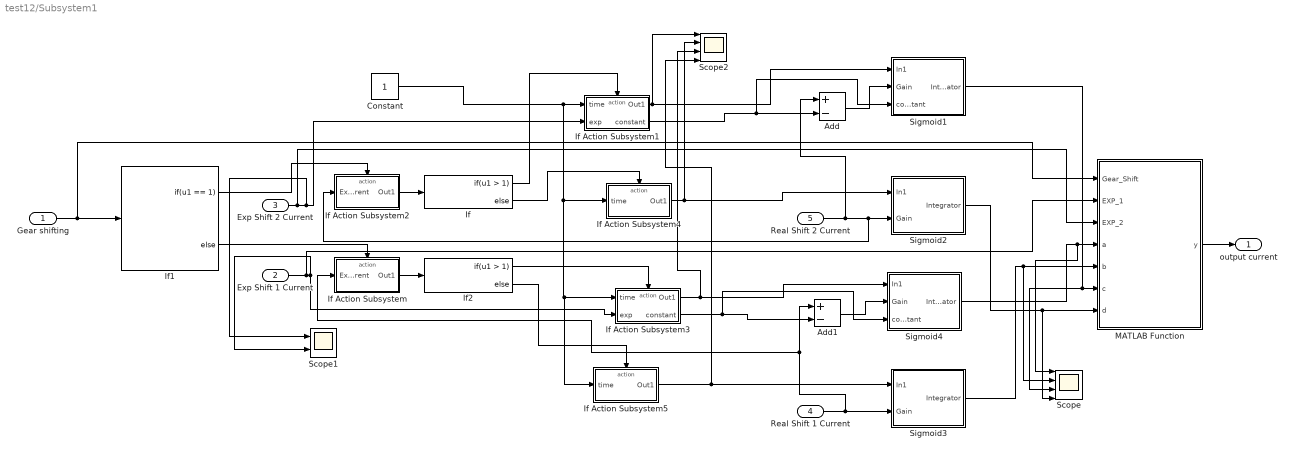
== system test12/Subsystem1 ==
  Gear shifting : Inport
  Exp Shift 1 Current : Inport  Port=2
  Exp Shift 2 Current : Inport  Port=3
  Real Shift 1 Current : Inport  Port=4
  Real Shift 2 Current : Inport  Port=5
  Add : Sum  Inputs=+-
  Add1 : Sum  Inputs=+-
  Constant : Constant
  If : If  IfExpression=u1 > 1
  If Action Subsystem : Subsystem  TreatAsAtomicUnit=on
  If Action Subsystem1 : Subsystem  TreatAsAtomicUnit=on
  If Action Subsystem2 : Subsystem  TreatAsAtomicUnit=on
  If Action Subsystem3 : Subsystem  TreatAsAtomicUnit=on
  If Action Subsystem4 : Subsystem  TreatAsAtomicUnit=on
  If Action Subsystem5 : Subsystem  TreatAsAtomicUnit=on
  If1 : If  IfExpression=u1 == 1
  If2 : If  IfExpression=u1 > 1
  MATLAB Function : MATLAB Function  TreatAsAtomicUnit=on
  Scope : Scope  NumInputPorts=4
  Scope1 : Scope  NumInputPorts=2
  Scope2 : Scope  NumInputPorts=4
  Sigmoid1 : Subsystem
  Sigmoid2 : Subsystem
  Sigmoid3 : Subsystem
  Sigmoid4 : Subsystem
  output current : Outport
  wires:
  Gear shifting/1 -> MATLAB Function/1(Gear_Shift), If1/1
  Real Shift 2 Current/1 -> Add/1, If Action Subsystem2/1(Exp Shift 2 Current), Sigmoid2/2(Gain)
  Real Shift 1 Current/1 -> If Action Subsystem/1(Exp Shift 1 Current), Add1/1, Sigmoid3/2(Gain)
  If1/1 -> If Action Subsystem2/Action
  If1/2 -> If Action Subsystem/Action
  Exp Shift 2 Current/1 -> MATLAB Function/3(EXP_2), Scope1/1, If Action Subsystem1/2(exp)
  Exp Shift 1 Current/1 -> MATLAB Function/2(EXP_1), If Action Subsystem3/2(exp), Scope1/2
  If Action Subsystem2/1(Out1) -> If/1
  If Action Subsystem/1(Out1) -> If2/1
  Constant/1 -> If Action Subsystem5/1(time), If Action Subsystem3/1(time), If Action Subsystem4/1(time), If Action Subsystem1/1(time)
  If Action Subsystem4/1(Out1) -> Scope2/2, Sigmoid2/1(In1)
  If Action Subsystem5/1(Out1) -> Scope2/4, Sigmoid3/1(In1)
  If Action Subsystem1/1(Out1) -> Scope2/1, Sigmoid1/1(In1)
  If Action Subsystem1/2(constant) -> Sigmoid1/3(constant), Add/2
  Add/1 -> Sigmoid1/2(Gain)
  If Action Subsystem3/1(Out1) -> Scope2/3, Sigmoid4/1(In1)
  Add1/1 -> Sigmoid4/2(Gain)
  If Action Subsystem3/2(constant) -> Sigmoid4/3(constant), Add1/2
  MATLAB Function/1(y) -> output current/1
  Sigmoid4/1(Integrator) -> Scope/1, MATLAB Function/4(a)
  Sigmoid3/1(Integrator) -> Scope/2, MATLAB Function/5(b)
  Sigmoid1/1(Integrator) -> MATLAB Function/6(c), Scope/3
  Sigmoid2/1(Integrator) -> MATLAB Function/7(d), Scope/4
  If2/1 -> If Action Subsystem3/Action
  If2/2 -> If Action Subsystem5/Action
  If/1 -> If Action Subsystem1/Action
  If/2 -> If Action Subsystem4/Action

== system test12/Clutch/RPM Sensor ==
  Mechanical Rotational Reference : fl_lib/Mechanical/Rotational Elements/Mechanical Rotational Reference
  Motion Sensor : fl_lib/Mechanical/Mechanical Sensors/Ideal Rotational Motion Sensor  reference=foundation.enum.MeasurementReference.difference  acceleration_port=false  velocity_port=true  position_port=true  wrap_angle=simscape.enum.onoff.off  offset=0 rad
  PS-Simulink Converter 2 : nesl_utility/PS-Simulink Converter  PhysicalDomain=network_engine_domain  SubClassName=ps_output  LeftPortType=input  RightPortType=output  PseudoPeriodic=off  Frequencies=[]  VectorFormat=1-D array  Unit=rpm  AffineConversion=off
  R : PMIOPort  Side=Left
  rpm : Outport  VectorParamsAs1DForOutWhenUnconnected=off
  wires:
  PS-Simulink Converter 2/1 -> rpm/1
  connections:
  R/RConn1 -- Motion Sensor/LConn1
  Motion Sensor/RConn1 -- Mechanical Rotational Reference/LConn1
  Motion Sensor/RConn2 -- PS-Simulink Converter 2/LConn1

== system test12/Clutch/RPM Sensor1 ==
  Mechanical Rotational Reference : fl_lib/Mechanical/Rotational Elements/Mechanical Rotational Reference
  Motion Sensor : fl_lib/Mechanical/Mechanical Sensors/Ideal Rotational Motion Sensor  reference=foundation.enum.MeasurementReference.difference  acceleration_port=false  velocity_port=true  position_port=true  wrap_angle=simscape.enum.onoff.off  offset=0 rad
  PS-Simulink Converter 2 : nesl_utility/PS-Simulink Converter  PhysicalDomain=network_engine_domain  SubClassName=ps_output  LeftPortType=input  RightPortType=output  PseudoPeriodic=off  Frequencies=[]  VectorFormat=1-D array  Unit=rpm  AffineConversion=off
  R : PMIOPort  Side=Left
  rpm : Outport  VectorParamsAs1DForOutWhenUnconnected=off
  wires:
  PS-Simulink Converter 2/1 -> rpm/1
  connections:
  R/RConn1 -- Motion Sensor/LConn1
  Motion Sensor/RConn1 -- Mechanical Rotational Reference/LConn1
  Motion Sensor/RConn2 -- PS-Simulink Converter 2/LConn1

== system test12/Clutch/Subsystem ==
  Last Output : Inport
  Input Current : Inport  Port=2
  Abs : Abs  SaturateOnIntegerOverflow=off
  Derivative : Derivative
  If Action Subsystem : Subsystem  TreatAsAtomicUnit=on
  If Action Subsystem1 : Subsystem  TreatAsAtomicUnit=on
  If1 : If  IfExpression=u1 <= 200
  Merge : Merge
  Scope : Scope  NumInputPorts=3
  Torque : Outport
  wires:
  Input Current/1 -> Scope/1, If Action Subsystem1/1(Input Current), Derivative/1
  If1/1 -> If Action Subsystem1/Action
  If1/2 -> If Action Subsystem/Action
  Last Output/1 -> Scope/2, If Action Subsystem/1(Last Output)
  If Action Subsystem1/1(Out1) -> Merge/1
  If Action Subsystem/1(Out1) -> Merge/2
  Merge/1 -> Scope/3, Torque/1
  Derivative/1 -> Abs/1  "I dot"
  Abs/1 -> If1/1

== system test12/Clutch/Subsystem2 ==
  Input Current : Inport
  Last Output : Inport  Port=2
  Abs : Abs  SaturateOnIntegerOverflow=off
  Derivative : Derivative
  If Action Subsystem : Subsystem  TreatAsAtomicUnit=on
  If Action Subsystem1 : Subsystem  TreatAsAtomicUnit=on
  If1 : If  IfExpression=u1 <= 200
  Merge : Merge
  Scope : Scope  NumInputPorts=3
  Torque : Outport
  wires:
  Input Current/1 -> Scope/1, If Action Subsystem1/1(Input Current), Derivative/1
  If1/1 -> If Action Subsystem1/Action
  If1/2 -> If Action Subsystem/Action
  Last Output/1 -> Scope/2, If Action Subsystem/1(Last Output)
  If Action Subsystem1/1(Out1) -> Merge/1
  If Action Subsystem/1(Out1) -> Merge/2
  Merge/1 -> Scope/3, Torque/1
  Derivative/1 -> Abs/1  "I dot"
  Abs/1 -> If1/1

== system test12/Gear Shifting Strategy/If Action Subsystem ==
  In1 : Inport
  Action Port : ActionPort  PropagateVarSize=During execution  ActionPortLabel=if(u1 == 2)
  Integrator : Integrator
  Out1 : Outport
  wires:
  In1/1 -> Integrator/1
  Integrator/1 -> Out1/1

== system test12/Gear Shifting Strategy/If Action Subsystem1 ==
  In1 : Inport
  Action Port : ActionPort  InitializeStates=reset  PropagateVarSize=During execution  ActionPortLabel=elseif(u1 == 1)
  Integrator : Integrator
  Out1 : Outport
  wires:
  In1/1 -> Integrator/1
  Integrator/1 -> Out1/1

== system test12/Gear Shifting Strategy/Sigmoid ==
  In1 : Inport
  Constant1 : Constant
  Constant2 : Constant  Value=-7.5
  Constant3 : Constant  Value=-1
  Gain : Gain  Gain=10
  Gain1 : Gain  Gain=100
  Math Function : Math  Operator=pow
  Math Function1 : Math
  Scope : Scope  NumInputPorts=2
  Sum : Sum  Inputs=|++
  Sum1 : Sum  Inputs=|++
  Integrator : Outport
  wires:
  Constant1/1 -> Sum1/1
  Sum1/1 -> Math Function/1
  Constant3/1 -> Math Function/2
  Sum/1 -> Math Function1/1
  Math Function/1 -> Gain/1
  Gain1/1 -> Sum/1
  Gain/1 -> Integrator/1, Scope/1
  Math Function1/1 -> Sum1/2
  Constant2/1 -> Sum/2
  In1/1 -> Gain1/1

== system test12/Gear Shifting Strategy/Sigmoid1 ==
  In1 : Inport
  Constant1 : Constant
  Constant2 : Constant  Value=-7.5
  Constant3 : Constant  Value=-1
  Gain : Gain  Gain=10
  Gain1 : Gain  Gain=100
  Math Function : Math  Operator=pow
  Math Function1 : Math
  Scope : Scope  NumInputPorts=2
  Sum : Sum  Inputs=|++
  Sum1 : Sum  Inputs=|++
  Integrator : Outport
  wires:
  Constant1/1 -> Sum1/1
  Sum1/1 -> Math Function/1
  Constant3/1 -> Math Function/2
  Sum/1 -> Math Function1/1
  Math Function/1 -> Gain/1
  Gain1/1 -> Sum/1
  Gain/1 -> Integrator/1, Scope/1
  Math Function1/1 -> Sum1/2
  Constant2/1 -> Sum/2
  In1/1 -> Gain1/1

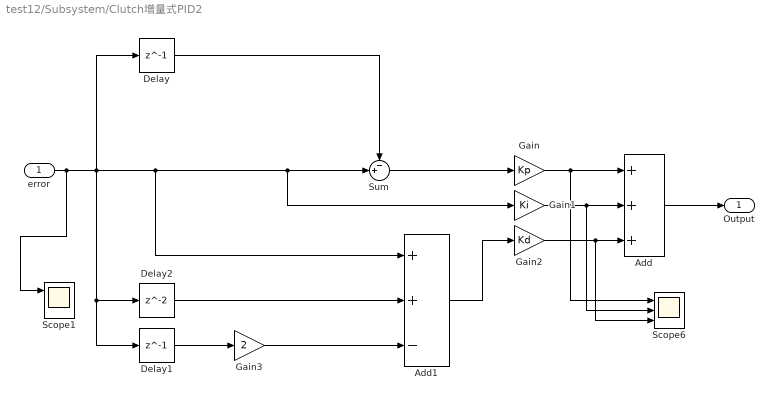
== system test12/Subsystem/Clutch增量式PID2 ==
  error : Inport
  Add : Sum  Inputs=+++
  Add1 : Sum  Inputs=++-
  Delay : Delay  DelayLength=1  InitialCondition=0
  Delay1 : Delay  DelayLength=1  InitialCondition=0
  Delay2 : Delay  InitialCondition=0
  Gain : Gain  Gain=Kp
  Gain1 : Gain  Gain=Ki
  Gain2 : Gain  Gain=Kd
  Gain3 : Gain  Gain=2
  Scope1 : Scope  NumInputPorts=3
  Scope6 : Scope  NumInputPorts=3
  Sum : Sum  Inputs=-+|
  Output : Outport
  wires:
  error/1 -> Scope1/1, Delay1/1, Delay2/1, Add1/1, Gain1/1, Sum/2, Delay/1
  Add/1 -> Output/1
  Gain2/1 -> Scope6/3, Add/3
  Gain1/1 -> Scope6/2, Add/2
  Gain/1 -> Scope6/1, Add/1
  Delay/1 -> Sum/1
  Sum/1 -> Gain/1
  Delay1/1 -> Gain3/1
  Gain3/1 -> Add1/3
  Delay2/1 -> Add1/2
  Add1/1 -> Gain2/1

== system test12/Subsystem/Motor增量式PID2 ==
  error : Inport
  Add : Sum  Inputs=+++
  Add1 : Sum  Inputs=++-
  Delay : Delay  DelayLength=1  InitialCondition=0
  Delay1 : Delay  DelayLength=1  InitialCondition=0
  Delay2 : Delay  InitialCondition=0
  Gain : Gain  Gain=Kp
  Gain1 : Gain  Gain=Ki
  Gain2 : Gain  Gain=Kd
  Gain3 : Gain  Gain=2
  Sum : Sum  Inputs=-+|
  Output : Outport
  wires:
  error/1 -> Delay1/1, Delay2/1, Add1/1, Gain1/1, Sum/2, Delay/1
  Add/1 -> Output/1
  Gain2/1 -> Add/3
  Gain1/1 -> Add/2
  Gain/1 -> Add/1
  Delay/1 -> Sum/1
  Sum/1 -> Gain/1
  Delay1/1 -> Gain3/1
  Gain3/1 -> Add1/3
  Delay2/1 -> Add1/2
  Add1/1 -> Gain2/1

== system test12/Subsystem/速度增量式PID ==
  error : Inport
  Add : Sum  Inputs=+++
  Add1 : Sum  Inputs=++-
  Delay : Delay  DelayLength=1  InitialCondition=0
  Delay1 : Delay  DelayLength=1  InitialCondition=0
  Delay2 : Delay  InitialCondition=0
  Gain : Gain  Gain=Kp
  Gain1 : Gain  Gain=Ki
  Gain2 : Gain  Gain=Kd
  Gain3 : Gain  Gain=2
  Sum : Sum  Inputs=-+|
  Output : Outport
  wires:
  error/1 -> Delay1/1, Delay2/1, Add1/1, Gain1/1, Sum/2, Delay/1
  Add/1 -> Output/1
  Gain2/1 -> Add/3
  Gain1/1 -> Add/2
  Gain/1 -> Add/1
  Delay/1 -> Sum/1
  Sum/1 -> Gain/1
  Delay1/1 -> Gain3/1
  Gain3/1 -> Add1/3
  Delay2/1 -> Add1/2
  Add1/1 -> Gain2/1

== system test12/Subsystem/速度增量式PID1 ==
  error : Inport
  Add : Sum  Inputs=+++
  Add1 : Sum  Inputs=++-
  Delay : Delay  DelayLength=1  InitialCondition=0
  Delay1 : Delay  DelayLength=1  InitialCondition=0
  Delay2 : Delay  InitialCondition=0
  Gain : Gain  Gain=Kp
  Gain1 : Gain  Gain=Ki
  Gain2 : Gain  Gain=Kd
  Gain3 : Gain  Gain=2
  Sum : Sum  Inputs=-+|
  Output : Outport
  wires:
  error/1 -> Delay1/1, Delay2/1, Add1/1, Gain1/1, Sum/2, Delay/1
  Add/1 -> Output/1
  Gain2/1 -> Add/3
  Gain1/1 -> Add/2
  Gain/1 -> Add/1
  Delay/1 -> Sum/1
  Sum/1 -> Gain/1
  Delay1/1 -> Gain3/1
  Gain3/1 -> Add1/3
  Delay2/1 -> Add1/2
  Add1/1 -> Gain2/1

== system test12/Subsystem1/If Action Subsystem ==
  Exp Shift 1 Current : Inport
  Action Port : ActionPort  InitializeStates=reset  ActionPortLabel=else
  Out1 : Outport
  wires:
  Exp Shift 1 Current/1 -> Out1/1

== system test12/Subsystem1/If Action Subsystem1 ==
  time : Inport
  exp : Inport  Port=2
  Action Port : ActionPort  InitializeStates=reset  PropagateVarSize=During execution  ActionPortLabel=if(u1 > 1)
  Integrator : Integrator
  Out1 : Outport
  constant : Outport  Port=2
  wires:
  time/1 -> Integrator/1
  exp/1 -> constant/1
  Integrator/1 -> Out1/1

== system test12/Subsystem1/If Action Subsystem2 ==
  Exp Shift 2 Current : Inport
  Action Port : ActionPort  InitializeStates=reset  PropagateVarSize=During execution  ActionPortLabel=if(u1 == 1)
  Out1 : Outport
  wires:
  Exp Shift 2 Current/1 -> Out1/1

== system test12/Subsystem1/If Action Subsystem3 ==
  time : Inport
  exp : Inport  Port=2
  Action Port : ActionPort  InitializeStates=reset  ActionPortLabel=if(u1 > 1)
  Integrator : Integrator
  Out1 : Outport
  constant : Outport  Port=2
  wires:
  time/1 -> Integrator/1
  exp/1 -> constant/1
  Integrator/1 -> Out1/1

== system test12/Subsystem1/If Action Subsystem4 ==
  time : Inport
  Action Port : ActionPort  InitializeStates=reset  PropagateVarSize=During execution  ActionPortLabel=else
  Integrator : Integrator
  Out1 : Outport
  wires:
  time/1 -> Integrator/1
  Integrator/1 -> Out1/1

== system test12/Subsystem1/If Action Subsystem5 ==
  time : Inport
  Action Port : ActionPort  InitializeStates=reset  ActionPortLabel=else
  Integrator : Integrator
  Out1 : Outport
  wires:
  time/1 -> Integrator/1
  Integrator/1 -> Out1/1

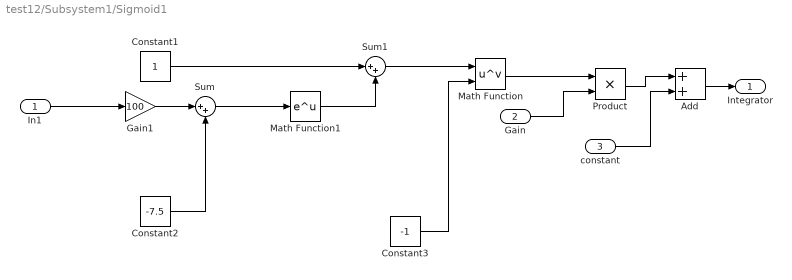
== system test12/Subsystem1/Sigmoid1 ==
  In1 : Inport
  Gain : Inport  Port=2
  constant : Inport  Port=3
  Add : Sum
  Constant1 : Constant
  Constant2 : Constant  Value=-7.5
  Constant3 : Constant  Value=-1
  Gain1 : Gain  Gain=100
  Math Function : Math  Operator=pow
  Math Function1 : Math
  Product : Product
  Sum : Sum  Inputs=|++
  Sum1 : Sum  Inputs=|++
  Integrator : Outport
  wires:
  Constant1/1 -> Sum1/1
  Sum1/1 -> Math Function/1
  Constant3/1 -> Math Function/2
  Sum/1 -> Math Function1/1
  Gain1/1 -> Sum/1
  Math Function1/1 -> Sum1/2
  Constant2/1 -> Sum/2
  In1/1 -> Gain1/1
  Math Function/1 -> Product/1
  Gain/1 -> Product/2
  Add/1 -> Integrator/1
  Product/1 -> Add/1
  constant/1 -> Add/2

== system test12/Subsystem1/Sigmoid2 ==
  In1 : Inport
  Gain : Inport  Port=2
  Constant1 : Constant
  Constant2 : Constant  Value=-7.5
  Constant3 : Constant  Value=-1
  Gain1 : Gain  Gain=100
  Math Function : Math  Operator=pow
  Math Function1 : Math
  Product : Product
  Sum : Sum  Inputs=|++
  Sum1 : Sum  Inputs=|++
  Integrator : Outport
  wires:
  Constant1/1 -> Sum1/1
  Sum1/1 -> Math Function/1
  Constant3/1 -> Math Function/2
  Sum/1 -> Math Function1/1
  Gain1/1 -> Sum/1
  Math Function1/1 -> Sum1/2
  Constant2/1 -> Sum/2
  In1/1 -> Gain1/1
  Math Function/1 -> Product/1
  Product/1 -> Integrator/1
  Gain/1 -> Product/2

== system test12/Subsystem1/Sigmoid3 ==
  In1 : Inport
  Gain : Inport  Port=2
  Constant1 : Constant
  Constant2 : Constant  Value=-7.5
  Constant3 : Constant  Value=-1
  Gain1 : Gain  Gain=100
  Math Function : Math  Operator=pow
  Math Function1 : Math
  Product : Product
  Sum : Sum  Inputs=|++
  Sum1 : Sum  Inputs=|++
  Integrator : Outport
  wires:
  Constant1/1 -> Sum1/1
  Sum1/1 -> Math Function/1
  Constant3/1 -> Math Function/2
  Sum/1 -> Math Function1/1
  Gain1/1 -> Sum/1
  Math Function1/1 -> Sum1/2
  Constant2/1 -> Sum/2
  In1/1 -> Gain1/1
  Math Function/1 -> Product/1
  Product/1 -> Integrator/1
  Gain/1 -> Product/2

== system test12/Subsystem1/Sigmoid4 ==
  In1 : Inport
  Gain : Inport  Port=2
  constant : Inport  Port=3
  Add : Sum
  Constant1 : Constant
  Constant2 : Constant  Value=-7.5
  Constant3 : Constant  Value=-1
  Gain1 : Gain  Gain=100
  Math Function : Math  Operator=pow
  Math Function1 : Math
  Product : Product
  Sum : Sum  Inputs=|++
  Sum1 : Sum  Inputs=|++
  Integrator : Outport
  wires:
  Constant1/1 -> Sum1/1
  Sum1/1 -> Math Function/1
  Constant3/1 -> Math Function/2
  Sum/1 -> Math Function1/1
  Gain1/1 -> Sum/1
  Math Function1/1 -> Sum1/2
  Constant2/1 -> Sum/2
  In1/1 -> Gain1/1
  Math Function/1 -> Product/1
  Gain/1 -> Product/2
  Add/1 -> Integrator/1
  Product/1 -> Add/1
  constant/1 -> Add/2

== system test12/Clutch/Subsystem/If Action Subsystem ==
  Last Output : Inport
  Action Port : ActionPort  PropagateVarSize=During execution  ActionPortLabel=else
  Out1 : Outport
  wires:
  Last Output/1 -> Out1/1

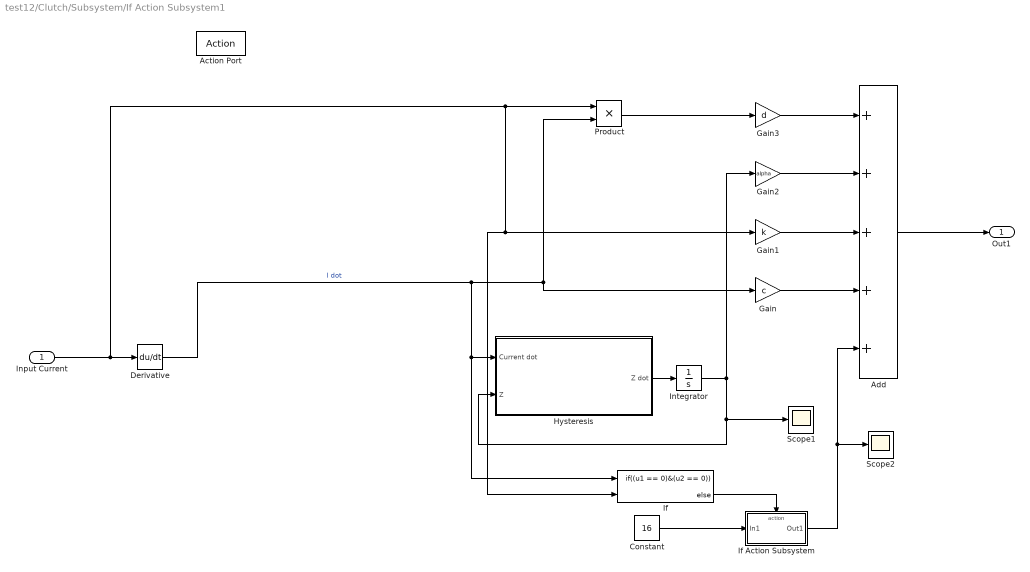
== system test12/Clutch/Subsystem/If Action Subsystem1 ==
  Input Current : Inport
  Action Port : ActionPort  InitializeStates=reset  PropagateVarSize=During execution  ActionPortLabel=if(u1 <= 200)
  Add : Sum  Inputs=+++++
  Constant : Constant  Value=16
  Derivative : Derivative
  Gain : Gain  Gain=c
  Gain1 : Gain  Gain=k
  Gain2 : Gain  Gain=alpha
  Gain3 : Gain  Gain=d
  Hysteresis : Subsystem  mask{theta=-0.41731, beta=-0.83796, v=2.2221, gamma=2.0211}
  If : If  NumInputs=2  IfExpression=(u1 == 0)&(u2 == 0)
  If Action Subsystem : Subsystem  TreatAsAtomicUnit=on
  Integrator : Integrator
  Product : Product
  Scope1 : Scope
  Scope2 : Scope
  Out1 : Outport
  wires:
  Gain1/1 -> Add/3
  Gain/1 -> Add/4
  Derivative/1 -> If/1, Hysteresis/1(Current dot), Product/2, Gain/1  "I dot"
  Product/1 -> Gain3/1
  Constant/1 -> If Action Subsystem/1(In1)
  If/2 -> If Action Subsystem/Action
  Add/1 -> Out1/1
  Hysteresis/1(Z dot) -> Integrator/1
  Input Current/1 -> If/2, Gain1/1, Product/1, Derivative/1
  Integrator/1 -> Scope1/1, Hysteresis/2(Z), Gain2/1
  Gain3/1 -> Add/1
  Gain2/1 -> Add/2
  If Action Subsystem/1(Out1) -> Scope2/1, Add/5

== system test12/Clutch/Subsystem2/If Action Subsystem ==
  Last Output : Inport
  Action Port : ActionPort  PropagateVarSize=During execution  ActionPortLabel=else
  Out1 : Outport
  wires:
  Last Output/1 -> Out1/1

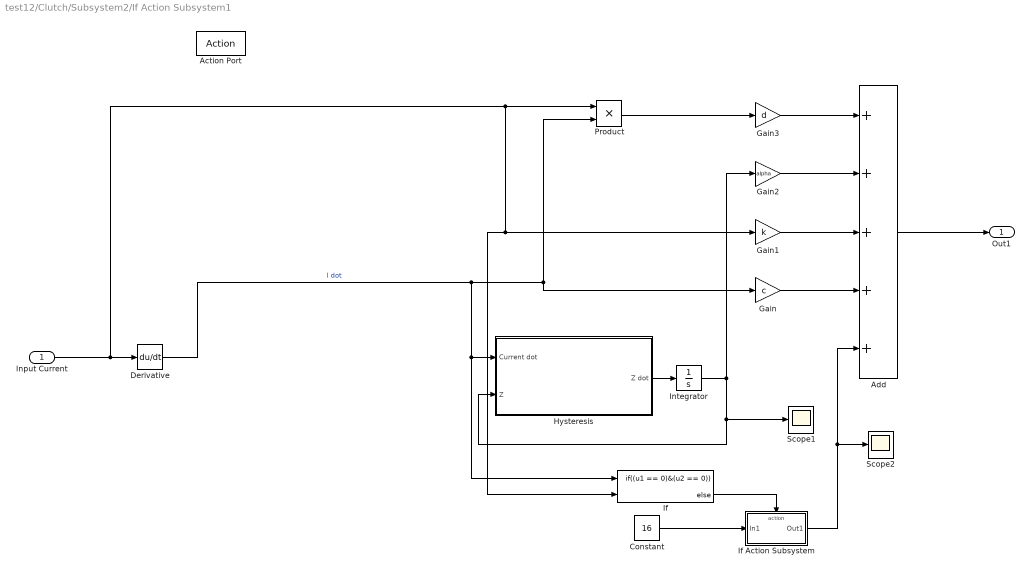
== system test12/Clutch/Subsystem2/If Action Subsystem1 ==
  Input Current : Inport
  Action Port : ActionPort  InitializeStates=reset  PropagateVarSize=During execution  ActionPortLabel=if(u1 <= 200)
  Add : Sum  Inputs=+++++
  Constant : Constant  Value=16
  Derivative : Derivative
  Gain : Gain  Gain=c
  Gain1 : Gain  Gain=k
  Gain2 : Gain  Gain=alpha
  Gain3 : Gain  Gain=d
  Hysteresis : Subsystem  mask{theta=-0.41731, beta=-0.83796, v=2.2221, gamma=2.0211}
  If : If  NumInputs=2  IfExpression=(u1 == 0)&(u2 == 0)
  If Action Subsystem : Subsystem  TreatAsAtomicUnit=on
  Integrator : Integrator
  Product : Product
  Scope1 : Scope
  Scope2 : Scope
  Out1 : Outport
  wires:
  Gain1/1 -> Add/3
  Gain/1 -> Add/4
  Derivative/1 -> If/1, Hysteresis/1(Current dot), Product/2, Gain/1  "I dot"
  Product/1 -> Gain3/1
  Constant/1 -> If Action Subsystem/1(In1)
  If/2 -> If Action Subsystem/Action
  Add/1 -> Out1/1
  Hysteresis/1(Z dot) -> Integrator/1
  Input Current/1 -> If/2, Gain1/1, Product/1, Derivative/1
  Integrator/1 -> Scope1/1, Hysteresis/2(Z), Gain2/1
  Gain3/1 -> Add/1
  Gain2/1 -> Add/2
  If Action Subsystem/1(Out1) -> Scope2/1, Add/5

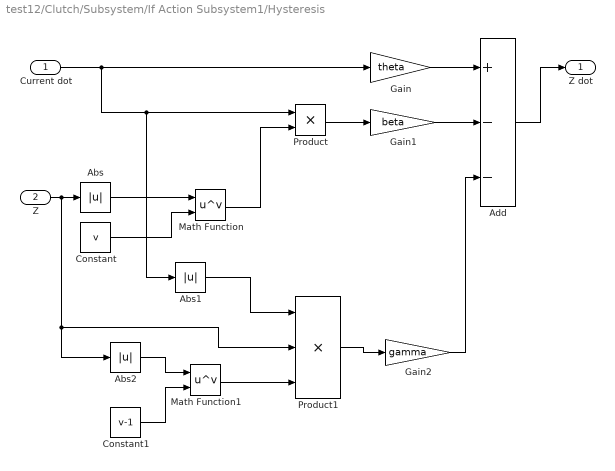
== system test12/Clutch/Subsystem/If Action Subsystem1/Hysteresis ==
  Current dot : Inport
  Z : Inport  Port=2
  Abs : Abs  SaturateOnIntegerOverflow=off
  Abs1 : Abs  SaturateOnIntegerOverflow=off
  Abs2 : Abs  SaturateOnIntegerOverflow=off
  Add : Sum  Inputs=+--
  Constant : Constant  Value=v
  Constant1 : Constant  Value=v-1
  Gain : Gain  Gain=theta
  Gain1 : Gain  Gain=beta
  Gain2 : Gain  Gain=gamma
  Math Function : Math  Operator=pow
  Math Function1 : Math  Operator=pow
  Product : Product
  Product1 : Product  Inputs=3
  Z dot : Outport
  wires:
  Current dot/1 -> Abs1/1, Product/1, Gain/1
  Gain/1 -> Add/1
  Z/1 -> Product1/2, Abs2/1, Abs/1
  Math Function/1 -> Product/2
  Product/1 -> Gain1/1
  Gain1/1 -> Add/2
  Math Function1/1 -> Product1/3
  Abs1/1 -> Product1/1
  Add/1 -> Z dot/1
  Abs/1 -> Math Function/1
  Constant/1 -> Math Function/2
  Product1/1 -> Gain2/1
  Gain2/1 -> Add/3
  Abs2/1 -> Math Function1/1
  Constant1/1 -> Math Function1/2

== system test12/Clutch/Subsystem/If Action Subsystem1/If Action Subsystem ==
  In1 : Inport
  Action Port : ActionPort  ActionPortLabel=else
  Out1 : Outport
  wires:
  In1/1 -> Out1/1

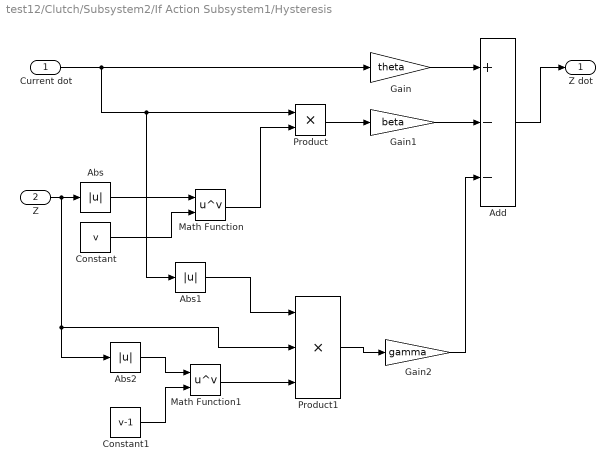
== system test12/Clutch/Subsystem2/If Action Subsystem1/Hysteresis ==
  Current dot : Inport
  Z : Inport  Port=2
  Abs : Abs  SaturateOnIntegerOverflow=off
  Abs1 : Abs  SaturateOnIntegerOverflow=off
  Abs2 : Abs  SaturateOnIntegerOverflow=off
  Add : Sum  Inputs=+--
  Constant : Constant  Value=v
  Constant1 : Constant  Value=v-1
  Gain : Gain  Gain=theta
  Gain1 : Gain  Gain=beta
  Gain2 : Gain  Gain=gamma
  Math Function : Math  Operator=pow
  Math Function1 : Math  Operator=pow
  Product : Product
  Product1 : Product  Inputs=3
  Z dot : Outport
  wires:
  Current dot/1 -> Abs1/1, Product/1, Gain/1
  Gain/1 -> Add/1
  Z/1 -> Product1/2, Abs2/1, Abs/1
  Math Function/1 -> Product/2
  Product/1 -> Gain1/1
  Gain1/1 -> Add/2
  Math Function1/1 -> Product1/3
  Abs1/1 -> Product1/1
  Add/1 -> Z dot/1
  Abs/1 -> Math Function/1
  Constant/1 -> Math Function/2
  Product1/1 -> Gain2/1
  Gain2/1 -> Add/3
  Abs2/1 -> Math Function1/1
  Constant1/1 -> Math Function1/2

== system test12/Clutch/Subsystem2/If Action Subsystem1/If Action Subsystem ==
  In1 : Inport
  Action Port : ActionPort  ActionPortLabel=else
  Out1 : Outport
  wires:
  In1/1 -> Out1/1

== matlab function test12/Subsystem1/MATLAB Function ==
  data: Gear_Shift input; y output; EXP_1 input; EXP_2 input; a input; b input; c input; d input
function y = fcn(Gear_Shift, EXP_1, EXP_2, a, b, c, d)

if Gear_Shift == 1
    if EXP_2 > 1
        y = a;
    else
        y = b;
    end
else
    if EXP_1 > 1
        y = c;
    else
        y = d;
    end
end

== matlab function test12/Subsystem/MATLAB Function1 ==
  data: u input; y output; Dead_Area input
function y = fcn(u,Dead_Area)

if (abs(u) >= Dead_Area) && (u< 0)
    y = -1*u ; 
elseif (abs(u) >= Dead_Area) && (u > 0)
       y = -1*u; 
else
 y = 0;
end

== matlab function test12/Subsystem/MATLAB Function2 ==
  data: u input; y output
function y = fcn(u)

if u < -10
    y = 10;
elseif u> 10
    y = 10;
else
   y = u;
end

== matlab function test12/Clutch/MATLAB Function1 ==
  data: boundary input; input_torque input; output_torque output
function output_torque = fcn(boundary, input_torque)

if boundary <= 0
    output_torque = 0;
else
    if abs(input_torque) <= boundary
        output_torque = input_torque;
    else
        if input_torque > 0
           output_torque = boundary;
        else
        output_torque = -1 * boundary;
        end
    end
end

== matlab function test12/Clutch/MATLAB Function2 ==
  data: boundary input; output_torque output; input_torque input
function output_torque = fcn(boundary, input_torque)

if boundary <= 0
    output_torque = 0;
else
    if abs(input_torque) <= boundary
        output_torque = input_torque;
    else
        if input_torque > 0
           output_torque = boundary;
        else
        output_torque = -1 * boundary;
        end
    end
end

== matlab function test12/Clutch/MATLAB Function ==
  data: Gear_1 input; Gear_Shifting output; Gear_2 input; Speed input
function Gear_Shifting = fcn(Gear_1, Gear_2, Speed)

if (Gear_2 > 4500)||(Speed > 60)
    Gear_Shifting = 2;
else
    Gear_Shifting = 1;
end
